simulink model "gm_hdl_generation_2"  (R2024b)
settings: Solver=VariableStepAuto  StartTime=0.0  StopTime=10.0  RelTol=1e-3
libraries: hdlmdlgenlib x4
settings Model: Creator=keybo  LastModifiedBy=keybo
settings OptimizationCC: BlockReduction=off  ConditionallyExecuteInputs=off  UseFloatMulNetSlope=on  InheritOutputTypeSmallerThanSingle=on  DefaultUnderspecifiedDataType=single
settings DebuggingCC: InheritedTsInSrcMsg=none

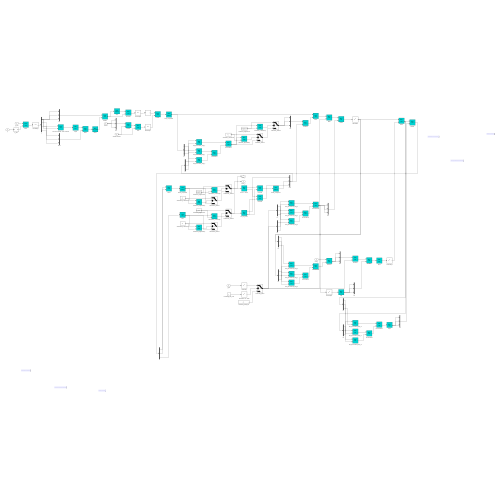
[thumbnail: Simulink's stored preview of the top-level diagram]
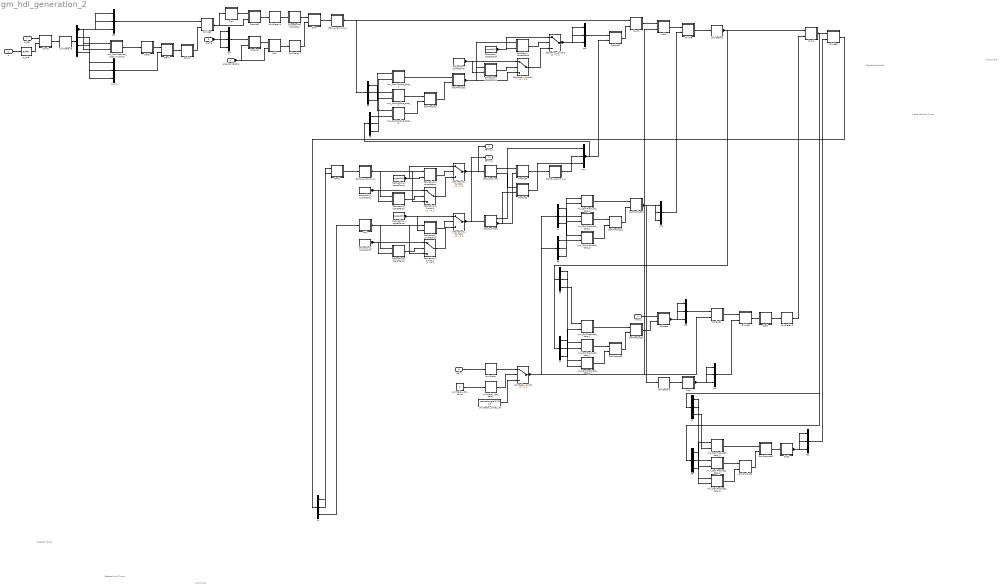
== system gm_hdl_generation_2 ==
  note: Attitude Controller
  note: Perpendicular Thrust
  note: Parallel Thrust
  note: Desired Unit Thrust
  note: Input to PID
  note: Unit Thrust
  q_des : Inport  OutDataTypeStr=single  PortDimensions=[4]  SampleTime=0.001
  q : Inport  Port=2  OutDataTypeStr=single  PortDimensions=[4]  SampleTime=0.001
  Inertia : Inport  Port=3  OutDataTypeStr=single  PortDimensions=1  SampleTime=0.001
  Angular Velocity : Inport  Port=4  OutDataTypeStr=single  PortDimensions=[3]  SampleTime=0.001
  r_gim : Inport  Port=5  OutDataTypeStr=single  PortDimensions=[3]  SampleTime=0.001
  norm_t : Inport  Port=6  OutDataTypeStr=single  PortDimensions=1  SampleTime=0.001
  Add : Subsystem
      mask Display: disp('NFP\nadd');
  Add1 : Subsystem
      mask Display: disp('NFP\nadd');
  Asin : Subsystem
      mask Display: disp('NFP\ntrig');
  Atan1 : Subsystem
      mask Display: disp('NFP\ntrig3');
  Atan2 : Subsystem
      mask Display: disp('NFP\ntrig3');
  Cos1_to_sincos : Subsystem
      mask Display: disp('NFP\ntrig2');
  Cos_to_sincos : Subsystem
      mask Display: disp('NFP\ntrig2');
  Discrete PID Controller : Subsystem
  Divide : Subsystem
      mask Display: disp('NFP\nmul');
  Divide1 : Subsystem
      mask Display: disp('NFP\nmul');
  Divide2 : Subsystem
      mask Display: disp('NFP\nmul');
  Divide3 : Subsystem
      mask Display: disp('NFP\nmul');
  Dot Product : Subsystem
      mask Display: disp('NFP\nadd');
  Dot Product1 : Subsystem
      mask Display: disp('NFP\nadd');
  Dot Product11 : Subsystem
      mask Display: disp('NFP\nadd');
  Dot Product12 : Subsystem
      mask Display: disp('NFP\nadd');
  Dot Product2 : Subsystem
      mask Display: disp('NFP\nadd');
  Dot Product21 : Subsystem
      mask Display: disp('NFP\nadd');
  Dot Product3 : Subsystem
      mask Display: disp('NFP\nadd');
  Dot Product31 : Subsystem
      mask Display: disp('NFP\nadd');
  Gain1 : Subsystem
      mask Display: disp('NFP\ngain_pow2');
  Gain2_unaryminus : Subsystem
      mask Display: disp('NFP\numinus');
  Gain3_unaryminus : Subsystem
      mask Display: disp('NFP\numinus');
  Gain_unaryminus : Subsystem
      mask Display: disp('NFP\numinus');
  Product : Subsystem
      mask Display: disp('NFP\nmul');
  Product1 : Subsystem
      mask Display: disp('NFP\nmul');
  Product2 : Subsystem
      mask Display: disp('NFP\nmul');
  Product3 : Subsystem
      mask Display: disp('NFP\nmul');
  Product4 : Subsystem
      mask Display: disp('NFP\nmul');
  Product5 : Subsystem
      mask Display: disp('NFP\nmul');
  Saturation1_LowerConst : Constant  Value=single(-0.5)  OutDataTypeStr=single  SampleTime=0.001
  Saturation1_LowerRelop : Subsystem
      mask Display: disp('NFP\nrelop');
  Saturation1_Switch1 : Switch  Criteria=u2 ~= 0  Threshold=double(0)  OutDataTypeStr=single  SampleTime=0.001  SaturateOnIntegerOverflow=off  InputSameDT=off
  Saturation1_Switch2 : Switch  Criteria=u2 ~= 0  Threshold=double(0)  OutDataTypeStr=single  SampleTime=0.001  SaturateOnIntegerOverflow=off  InputSameDT=off
  Saturation1_UpperConst : Constant  Value=single(0.5)  OutDataTypeStr=single  SampleTime=0.001
  Saturation1_UpperRelop : Subsystem
      mask Display: disp('NFP\nrelop');
  Saturation2_LowerConst : Constant  Value=single(-0.5)  OutDataTypeStr=single  SampleTime=0.001
  Saturation2_LowerRelop : Subsystem
      mask Display: disp('NFP\nrelop');
  Saturation2_Switch1 : Switch  Criteria=u2 ~= 0  Threshold=double(0)  OutDataTypeStr=single  SampleTime=0.001  SaturateOnIntegerOverflow=off  InputSameDT=off
  Saturation2_Switch2 : Switch  Criteria=u2 ~= 0  Threshold=double(0)  OutDataTypeStr=single  SampleTime=0.001  SaturateOnIntegerOverflow=off  InputSameDT=off
  Saturation2_UpperConst : Constant  Value=single(0.5)  OutDataTypeStr=single  SampleTime=0.001
  Saturation2_UpperRelop : Subsystem
      mask Display: disp('NFP\nrelop');
  Saturation_LowerConst : Constant  Value=single(-0.5)  OutDataTypeStr=single  SampleTime=0.001
  Saturation_LowerRelop : Subsystem
      mask Display: disp('NFP\nrelop');
  Saturation_Switch1 : Switch  Criteria=u2 ~= 0  Threshold=double(0)  OutDataTypeStr=single  SampleTime=0.001  SaturateOnIntegerOverflow=off  InputSameDT=off
  Saturation_Switch2 : Switch  Criteria=u2 ~= 0  Threshold=double(0)  OutDataTypeStr=single  SampleTime=0.001  SaturateOnIntegerOverflow=off  InputSameDT=off
  Saturation_UpperConst : Constant  Value=single(0.5)  OutDataTypeStr=single  SampleTime=0.001
  Saturation_UpperRelop : Subsystem
      mask Display: disp('NFP\nrelop');
  Sign : Subsystem
      mask Display: disp('NFP\nsignum');
  Sqrt : Subsystem
      mask Display: disp('NFP\nsqrt');
  Sqrt1 : Subsystem
      mask Display: disp('NFP\nsqrt');
  Sqrt2 : Subsystem
      mask Display: disp('NFP\nsqrt');
  Sqrt3 : Subsystem
      mask Display: disp('NFP\nsqrt');
  Subtract : Subsystem
      mask Display: disp('NFP\nadd');
  Sum : Subsystem
      mask Display: disp('NFP\nadd');
  Sum1 : Subsystem
      mask Display: disp('NFP\nadd');
  Sum2 : Subsystem
      mask Display: disp('NFP\nadd');
  Sum3 : Subsystem
      mask Display: disp('NFP\nadd');
  Unit Delay{,1..3,5..7} (7 alike) : Delay  DelayLength=double(1)  InitialCondition=0  SampleTime=0.001
  Unit Delay_Initial_Val : Constant  Value="repmat(single(1),[3  1])"  OutDataTypeStr=single  SampleTime=0.001
  Unit Delay_ctrl_const : Constant  OutDataTypeStr=boolean  SampleTime=0.001
  Unit Delay_ctrl_delay : Delay  DelayLength=double(1)  InitialCondition=0  SampleTime=0.001
  Unit Delay_switch : Switch  Criteria=u2 ~= 0  Threshold=double(0)  OutDataTypeStr=single  SampleTime=0.001  SaturateOnIntegerOverflow=off  InputSameDT=off
  mul_Dot Product1_dotp_0 : Subsystem
      mask Display: disp('NFP\nmul');
  mul_Dot Product1_dotp_1 : Subsystem
      mask Display: disp('NFP\nmul');
  mul_Dot Product1_dotp_2 : Subsystem
      mask Display: disp('NFP\nmul');
  mul_Dot Product2_dotp_0 : Subsystem
      mask Display: disp('NFP\nmul');
  mul_Dot Product2_dotp_1 : Subsystem
      mask Display: disp('NFP\nmul');
  mul_Dot Product2_dotp_2 : Subsystem
      mask Display: disp('NFP\nmul');
  mul_Dot Product3_dotp_0 : Subsystem
      mask Display: disp('NFP\nmul');
  mul_Dot Product3_dotp_1 : Subsystem
      mask Display: disp('NFP\nmul');
  mul_Dot Product3_dotp_2 : Subsystem
      mask Display: disp('NFP\nmul');
  mul_Dot Product4_dotp_mulcomp : Subsystem
      mask Display: disp('NFP\nmul');
  mul_Dot Product_dotp_0 : Subsystem
      mask Display: disp('NFP\nmul');
  mul_Dot Product_dotp_1 : Subsystem
      mask Display: disp('NFP\nmul');
  mul_Dot Product_dotp_2 : Subsystem
      mask Display: disp('NFP\nmul');
  mux : Mux  Inputs=3
  mux1 : Mux  Inputs=3
  q_wire : hdlmdlgenlib/Buffer
  t : Demux
  t{1..9} (9 alike) : Demux  Outputs=3
  t{10..16} (7 alike) : Mux  Inputs=3
  servo_x : Outport  SampleTime=0.001  VectorParamsAs1DForOutWhenUnconnected=off
  servo_y : Outport  Port=2  SampleTime=0.001  VectorParamsAs1DForOutWhenUnconnected=off
  wires:
  mul_Dot Product1_dotp_1/1(Out1) -> Dot Product11/1(In1)
  Dot Product31/1(Out1) -> Sqrt2/1(In1)
  t/3 -> mux1/2
  Saturation1_LowerRelop/1(Out1) -> Saturation1_Switch2/2
  Product3/1(Out1) -> Unit Delay6/1
  Unit Delay_switch/1 -> t4/1, t5/1, Product1/2(In2), Add1/2(In2)
  Discrete PID Controller/1(y) -> Sum/1(In1)
  Sqrt/1(Out1) -> t11/1, t11/2, t11/3
  t2/1 -> mul_Dot Product_dotp_0/1(In1)
  r_gim/1 -> Unit Delay/1
  Divide3/1(Out1) -> Sign/1(In1), Product3/2(In2)
  Dot Product2/1(Out1) -> Dot Product21/2(In2)
  Saturation2_UpperRelop/1(Out1) -> Saturation2_Switch1/2
  t2/3 -> mul_Dot Product_dotp_2/1(In1)
  Unit Delay_ctrl_delay/1 -> Unit Delay_switch/2
  t4/2 -> mul_Dot Product1_dotp_1/1(In1)
  Unit Delay_ctrl_const/1 -> Unit Delay_ctrl_delay/1
  t6/3 -> mul_Dot Product2_dotp_2/1(In1)
  Saturation2_UpperConst/1 -> Saturation2_LowerRelop/2(In2), Saturation2_Switch2/1
  mul_Dot Product2_dotp_1/1(Out1) -> Dot Product2/1(In1)
  Saturation2_LowerConst/1 -> Saturation2_UpperRelop/2(In2), Saturation2_Switch1/1
  Unit Delay3/1 -> Sum1/2(In2)
  Cos_to_sincos/1(Out1) -> mux/1
  t1/1 -> Atan2/1(In1)
  Unit Delay_Initial_Val/1 -> Unit Delay_switch/3
  t2/2 -> mul_Dot Product_dotp_1/1(In1)
  t1/2 -> Atan2/2(In2)
  t/4 -> mux1/3
  Cos_to_sincos/2(Out2) -> Product5/2(In2), Product4/2(In2)
  Dot Product11/1(Out1) -> Dot Product12/2(In2)
  mul_Dot Product3_dotp_0/1(Out1) -> Dot Product3/2(In2)
  Unit Delay2/1 -> Sqrt/1(In1)
  t/2 -> mux1/1
  t3/1 -> mul_Dot Product_dotp_0/2(In2)
  Sum2/1(Out1) -> Add1/1(In1)
  t4/3 -> mul_Dot Product1_dotp_2/1(In1)
  q_wire/1 -> Sum3/2(In2)
  Saturation1_Switch2/1 -> Cos1_to_sincos/1(In1), servo_x/1
  Sign/1(Out1) -> Product3/1(In1)
  Inertia/1 -> t14/1, t14/2, t14/3
  Dot Product12/1(Out1) -> t10/2, Unit Delay2/1, t10/1, t10/3
  Sum1/1(Out1) -> Divide2/1(In1), t9/1, t8/1
  t3/3 -> mul_Dot Product_dotp_2/2(In2)
  t3/2 -> mul_Dot Product_dotp_1/2(In2)
  t5/1 -> mul_Dot Product1_dotp_0/2(In2)
  t4/1 -> mul_Dot Product1_dotp_0/1(In1)
  Product5/1(Out1) -> mux/3
  t11/1 -> Divide1/2(In2)
  Sqrt3/1(Out1) -> Atan1/1(In1)
  norm_t/1 -> Subtract/1(In1)
  mul_Dot Product_dotp_2/1(Out1) -> Dot Product1/1(In1)
  Unit Delay1/1 -> Sum1/1(In1), t7/1, t6/1
  mul_Dot Product3_dotp_1/1(Out1) -> Dot Product3/1(In1)
  t8/2 -> mul_Dot Product3_dotp_1/1(In1)
  Add/1(Out1) -> Unit Delay7/1
  mul_Dot Product1_dotp_2/1(Out1) -> Dot Product12/1(In1)
  t16/1 -> Product2/1(In1)
  Sqrt2/1(Out1) -> t12/1, t12/2, t12/3
  Saturation_UpperConst/1 -> Saturation_LowerRelop/2(In2), Saturation_Switch2/1
  Saturation1_Switch1/1 -> Saturation1_Switch2/3
  Dot Product1/1(Out1) -> Saturation_Switch1/3, Saturation_UpperRelop/1(In1), Saturation_LowerRelop/1(In1)
  Gain_unaryminus/1(Out1) -> t2/1, Sum2/1(In1)
  Saturation_Switch1/1 -> Saturation_Switch2/3
  Angular Velocity/1 -> Product/2(In2), Add/2(In2)
  mul_Dot Product2_dotp_2/1(Out1) -> Dot Product21/1(In1)
  Saturation1_LowerConst/1 -> Saturation1_UpperRelop/2(In2), Saturation1_Switch1/1
  t1/3 -> Asin/1(In1)
  t6/2 -> mul_Dot Product2_dotp_1/1(In1)
  Sum3/1(Out1) -> Unit Delay5/1
  mux1/1 -> Atan1/2(In2)
  q/1 -> q_wire/1
  t8/3 -> mul_Dot Product3_dotp_2/1(In1)
  mux/1 -> Product2/2(In2), t3/1
  Gain2_unaryminus/1(Out1) -> Saturation1_UpperRelop/1(In1), Saturation1_LowerRelop/1(In1), Saturation1_Switch1/3
  t9/1 -> mul_Dot Product3_dotp_0/2(In2)
  Dot Product3/1(Out1) -> Dot Product31/2(In2)
  Asin/1(Out1) -> Saturation2_UpperRelop/1(In1), Saturation2_Switch1/3, Saturation2_LowerRelop/1(In1)
  Saturation1_UpperConst/1 -> Saturation1_LowerRelop/2(In2), Saturation1_Switch2/1
  Unit Delay7/1 -> Sum/2(In2)
  Saturation2_LowerRelop/1(Out1) -> Saturation2_Switch2/2
  Product2/1(Out1) -> Sum2/2(In2)
  Cos1_to_sincos/1(Out1) -> Product4/1(In1)
  Unit Delay5/1 -> t/1
  Divide1/1(Out1) -> Sqrt1/1(In1)
  Atan1/1(Out1) -> Gain1/1(In1)
  mul_Dot Product_dotp_1/1(Out1) -> Dot Product/1(In1)
  Gain3_unaryminus/1(Out1) -> mux/2
  Saturation2_Switch2/1 -> servo_y/1, Cos_to_sincos/1(In1)
  Gain1/1(Out1) -> Divide3/2(In2)
  mul_Dot Product4_dotp_mulcomp/1(Out1) -> Sqrt3/1(In1)
  Saturation_LowerConst/1 -> Saturation_UpperRelop/2(In2), Saturation_Switch1/1
  t5/3 -> mul_Dot Product1_dotp_2/2(In2)
  mul_Dot Product3_dotp_2/1(Out1) -> Dot Product31/1(In1)
  t14/1 -> Product/1(In1)
  mul_Dot Product_dotp_0/1(Out1) -> Dot Product/2(In2)
  Saturation2_Switch1/1 -> Saturation2_Switch2/3
  t8/1 -> mul_Dot Product3_dotp_0/1(In1)
  q_des/1 -> Sum3/1(In1)
  Dot Product21/1(Out1) -> Subtract/2(In2)
  Sum/1(Out1) -> Gain_unaryminus/1(In1)
  t9/3 -> mul_Dot Product3_dotp_2/2(In2)
  t/1 -> mul_Dot Product4_dotp_mulcomp/1(In1), t13/2, t13/1, t13/3, mul_Dot Product4_dotp_mulcomp/2(In2)
  Dot Product/1(Out1) -> Dot Product1/2(In2)
  t13/1 -> Divide3/1(In1)
  Saturation1_UpperRelop/1(Out1) -> Saturation1_Switch1/2
  t6/1 -> mul_Dot Product2_dotp_0/1(In1)
  Saturation_LowerRelop/1(Out1) -> Saturation_Switch2/2
  Divide2/1(Out1) -> t1/1
  Atan2/1(Out1) -> Gain2_unaryminus/1(In1)
  t9/2 -> mul_Dot Product3_dotp_1/2(In2)
  Product/1(Out1) -> Add/1(In1)
  Subtract/1(Out1) -> t15/1, t15/2, t15/3
  Cos1_to_sincos/2(Out2) -> Product5/1(In1)
  t5/2 -> mul_Dot Product1_dotp_1/2(In2)
  t7/2 -> mul_Dot Product2_dotp_1/2(In2)
  Unit Delay6/1 -> Discrete PID Controller/1(u)
  Saturation_Switch2/1 -> t16/1, t16/3, t16/2
  Sqrt1/1(Out1) -> Unit Delay3/1
  Product1/1(Out1) -> Divide1/1(In1)
  t7/1 -> mul_Dot Product2_dotp_0/2(In2)
  mul_Dot Product2_dotp_0/1(Out1) -> Dot Product2/2(In2)
  Unit Delay/1 -> Unit Delay_switch/1
  Divide/1(Out1) -> Unit Delay1/1
  t10/1 -> Divide/2(In2)
  t7/3 -> mul_Dot Product2_dotp_2/2(In2)
  Add1/1(Out1) -> Divide/1(In1)
  Saturation_UpperRelop/1(Out1) -> Saturation_Switch1/2
  t12/1 -> Divide2/2(In2)
  t15/1 -> Product1/1(In1)
  mul_Dot Product1_dotp_0/1(Out1) -> Dot Product11/2(In2)
  Product4/1(Out1) -> Gain3_unaryminus/1(In1)

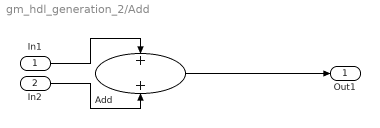
== system gm_hdl_generation_2/Add ==
  In1 : Inport
  In2 : Inport  Port=2
  Add : Sum  OutDataTypeStr=single  SampleTime=0.001
  Out1 : Outport
  wires:
  In1/1 -> Add/1
  In2/1 -> Add/2
  Add/1 -> Out1/1

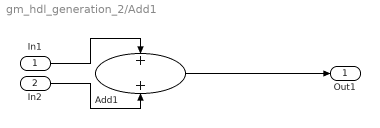
== system gm_hdl_generation_2/Add1 ==
  In1 : Inport
  In2 : Inport  Port=2
  Add1 : Sum  OutDataTypeStr=single  SampleTime=0.001
  Out1 : Outport
  wires:
  In1/1 -> Add1/1
  In2/1 -> Add1/2
  Add1/1 -> Out1/1

== system gm_hdl_generation_2/Asin ==
  In1 : Inport
  Asin : Trigonometry  Operator=asin  SampleTime=0.001
  Out1 : Outport
  wires:
  In1/1 -> Asin/1
  Asin/1 -> Out1/1

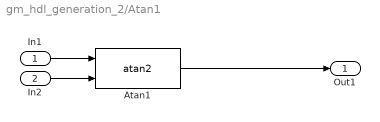
== system gm_hdl_generation_2/Atan1 ==
  In1 : Inport
  In2 : Inport  Port=2
  Atan1 : Trigonometry  Operator=atan2  SampleTime=0.001
  Out1 : Outport
  wires:
  In1/1 -> Atan1/1
  In2/1 -> Atan1/2
  Atan1/1 -> Out1/1

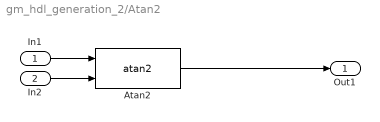
== system gm_hdl_generation_2/Atan2 ==
  In1 : Inport
  In2 : Inport  Port=2
  Atan2 : Trigonometry  Operator=atan2  SampleTime=0.001
  Out1 : Outport
  wires:
  In1/1 -> Atan2/1
  In2/1 -> Atan2/2
  Atan2/1 -> Out1/1

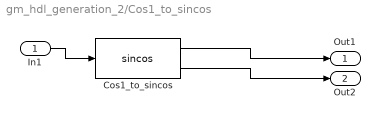
== system gm_hdl_generation_2/Cos1_to_sincos ==
  In1 : Inport
  Cos1_to_sincos : Trigonometry  Operator=sincos  SampleTime=0.001
  Out1 : Outport
  Out2 : Outport  Port=2
  wires:
  In1/1 -> Cos1_to_sincos/1
  Cos1_to_sincos/1 -> Out1/1
  Cos1_to_sincos/2 -> Out2/1

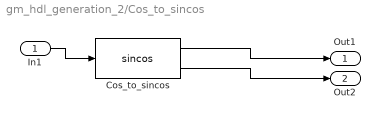
== system gm_hdl_generation_2/Cos_to_sincos ==
  In1 : Inport
  Cos_to_sincos : Trigonometry  Operator=sincos  SampleTime=0.001
  Out1 : Outport
  Out2 : Outport  Port=2
  wires:
  In1/1 -> Cos_to_sincos/1
  Cos_to_sincos/1 -> Out1/1
  Cos_to_sincos/2 -> Out2/1

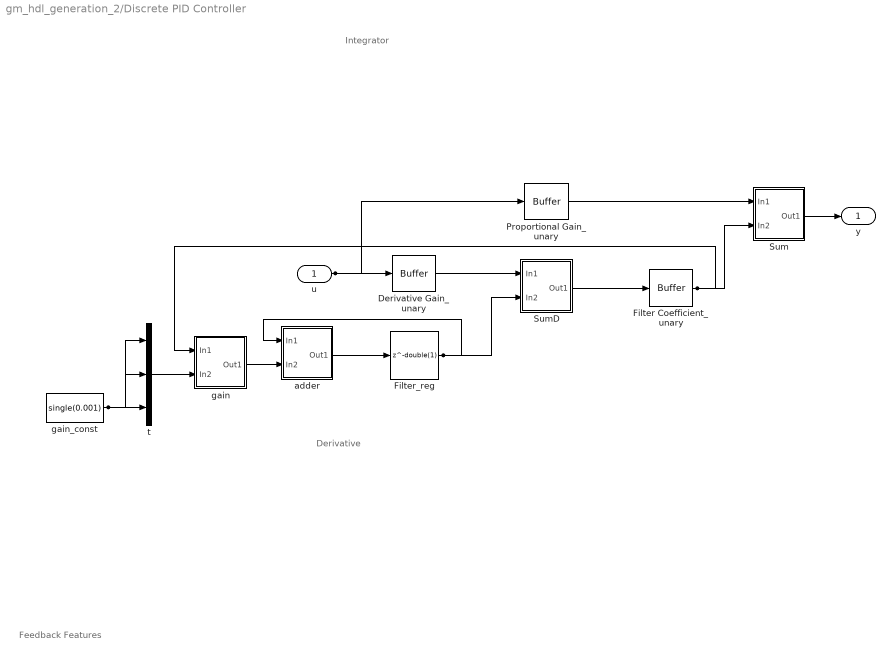
== system gm_hdl_generation_2/Discrete PID Controller ==
  note: Integrator
  note: Derivative
  note: Feedback Features
  u : Inport  OutDataTypeStr=single  PortDimensions=[3]  SampleTime=0.001
  Derivative Gain_unary : hdlmdlgenlib/Buffer
  Filter Coefficient_unary : hdlmdlgenlib/Buffer
  Filter_reg : Delay  DelayLength=double(1)  InitialCondition=0  SampleTime=0.001
  Proportional Gain_unary : hdlmdlgenlib/Buffer
  Sum : Subsystem
      mask Display: disp('NFP\nadd');
  SumD : Subsystem
      mask Display: disp('NFP\nadd');
  adder : Subsystem
      mask Display: disp('NFP\nadd');
  gain : Subsystem
      mask Display: disp('NFP\nmul');
  gain_const : Constant  Value=single(0.001)  OutDataTypeStr=single  SampleTime=0.001
  t : Mux  Inputs=3
  y : Outport  SampleTime=0.001
  wires:
  Filter Coefficient_unary/1 -> Sum/2(In2), gain/1(In1)
  Proportional Gain_unary/1 -> Sum/1(In1)
  Filter_reg/1 -> SumD/2(In2), adder/1(In1)
  Derivative Gain_unary/1 -> SumD/1(In1)
  adder/1(Out1) -> Filter_reg/1
  gain/1(Out1) -> adder/2(In2)
  SumD/1(Out1) -> Filter Coefficient_unary/1
  t/1 -> gain/2(In2)
  Sum/1(Out1) -> y/1
  u/1 -> Derivative Gain_unary/1, Proportional Gain_unary/1
  gain_const/1 -> t/1, t/2, t/3

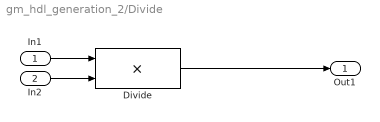
== system gm_hdl_generation_2/Divide ==
  In1 : Inport
  In2 : Inport  Port=2
  Divide : Product  Inputs=**  OutDataTypeStr=single  SampleTime=0.001
  Out1 : Outport
  wires:
  In1/1 -> Divide/1
  In2/1 -> Divide/2
  Divide/1 -> Out1/1

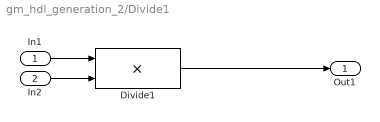
== system gm_hdl_generation_2/Divide1 ==
  In1 : Inport
  In2 : Inport  Port=2
  Divide1 : Product  Inputs=**  OutDataTypeStr=single  SampleTime=0.001
  Out1 : Outport
  wires:
  In1/1 -> Divide1/1
  In2/1 -> Divide1/2
  Divide1/1 -> Out1/1

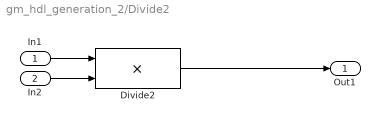
== system gm_hdl_generation_2/Divide2 ==
  In1 : Inport
  In2 : Inport  Port=2
  Divide2 : Product  Inputs=**  OutDataTypeStr=single  SampleTime=0.001
  Out1 : Outport
  wires:
  In1/1 -> Divide2/1
  In2/1 -> Divide2/2
  Divide2/1 -> Out1/1

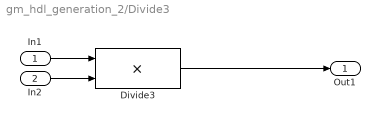
== system gm_hdl_generation_2/Divide3 ==
  In1 : Inport
  In2 : Inport  Port=2
  Divide3 : Product  Inputs=**  OutDataTypeStr=single  SampleTime=0.001
  Out1 : Outport
  wires:
  In1/1 -> Divide3/1
  In2/1 -> Divide3/2
  Divide3/1 -> Out1/1

== system gm_hdl_generation_2/Dot Product ==
  In1 : Inport
  In2 : Inport  Port=2
  Dot Product : Sum  OutDataTypeStr=single  SampleTime=0.001
  Out1 : Outport
  wires:
  In1/1 -> Dot Product/1
  In2/1 -> Dot Product/2
  Dot Product/1 -> Out1/1

== system gm_hdl_generation_2/Dot Product1 ==
  In1 : Inport
  In2 : Inport  Port=2
  Dot Product1 : Sum  OutDataTypeStr=single  SampleTime=0.001
  Out1 : Outport
  wires:
  In1/1 -> Dot Product1/1
  In2/1 -> Dot Product1/2
  Dot Product1/1 -> Out1/1

== system gm_hdl_generation_2/Dot Product11 ==
  In1 : Inport
  In2 : Inport  Port=2
  Dot Product11 : Sum  OutDataTypeStr=single  SampleTime=0.001
  Out1 : Outport
  wires:
  In1/1 -> Dot Product11/1
  In2/1 -> Dot Product11/2
  Dot Product11/1 -> Out1/1

== system gm_hdl_generation_2/Dot Product12 ==
  In1 : Inport
  In2 : Inport  Port=2
  Dot Product12 : Sum  OutDataTypeStr=single  SampleTime=0.001
  Out1 : Outport
  wires:
  In1/1 -> Dot Product12/1
  In2/1 -> Dot Product12/2
  Dot Product12/1 -> Out1/1

== system gm_hdl_generation_2/Dot Product2 ==
  In1 : Inport
  In2 : Inport  Port=2
  Dot Product2 : Sum  OutDataTypeStr=single  SampleTime=0.001
  Out1 : Outport
  wires:
  In1/1 -> Dot Product2/1
  In2/1 -> Dot Product2/2
  Dot Product2/1 -> Out1/1

== system gm_hdl_generation_2/Dot Product21 ==
  In1 : Inport
  In2 : Inport  Port=2
  Dot Product21 : Sum  OutDataTypeStr=single  SampleTime=0.001
  Out1 : Outport
  wires:
  In1/1 -> Dot Product21/1
  In2/1 -> Dot Product21/2
  Dot Product21/1 -> Out1/1

== system gm_hdl_generation_2/Dot Product3 ==
  In1 : Inport
  In2 : Inport  Port=2
  Dot Product3 : Sum  OutDataTypeStr=single  SampleTime=0.001
  Out1 : Outport
  wires:
  In1/1 -> Dot Product3/1
  In2/1 -> Dot Product3/2
  Dot Product3/1 -> Out1/1

== system gm_hdl_generation_2/Dot Product31 ==
  In1 : Inport
  In2 : Inport  Port=2
  Dot Product31 : Sum  OutDataTypeStr=single  SampleTime=0.001
  Out1 : Outport
  wires:
  In1/1 -> Dot Product31/1
  In2/1 -> Dot Product31/2
  Dot Product31/1 -> Out1/1

== system gm_hdl_generation_2/Gain1 ==
  In1 : Inport
  Gain1 : Gain  Gain=single(2)
  Out1 : Outport
  wires:
  In1/1 -> Gain1/1
  Gain1/1 -> Out1/1

== system gm_hdl_generation_2/Gain2_unaryminus ==
  In1 : Inport
  Gain2_unaryminus : UnaryMinus  SampleTime=0.001
  Out1 : Outport
  wires:
  In1/1 -> Gain2_unaryminus/1
  Gain2_unaryminus/1 -> Out1/1

== system gm_hdl_generation_2/Gain3_unaryminus ==
  In1 : Inport
  Gain3_unaryminus : UnaryMinus  SampleTime=0.001
  Out1 : Outport
  wires:
  In1/1 -> Gain3_unaryminus/1
  Gain3_unaryminus/1 -> Out1/1

== system gm_hdl_generation_2/Gain_unaryminus ==
  In1 : Inport
  Gain_unaryminus : UnaryMinus  SampleTime=0.001
  Out1 : Outport
  wires:
  In1/1 -> Gain_unaryminus/1
  Gain_unaryminus/1 -> Out1/1

== system gm_hdl_generation_2/Product ==
  In1 : Inport
  In2 : Inport  Port=2
  Product : Product  Inputs=**  OutDataTypeStr=single  SampleTime=0.001
  Out1 : Outport
  wires:
  In1/1 -> Product/1
  In2/1 -> Product/2
  Product/1 -> Out1/1

== system gm_hdl_generation_2/Product1 ==
  In1 : Inport
  In2 : Inport  Port=2
  Product1 : Product  Inputs=**  OutDataTypeStr=single  SampleTime=0.001
  Out1 : Outport
  wires:
  In1/1 -> Product1/1
  In2/1 -> Product1/2
  Product1/1 -> Out1/1

== system gm_hdl_generation_2/Product2 ==
  In1 : Inport
  In2 : Inport  Port=2
  Product2 : Product  Inputs=**  OutDataTypeStr=single  SampleTime=0.001
  Out1 : Outport
  wires:
  In1/1 -> Product2/1
  In2/1 -> Product2/2
  Product2/1 -> Out1/1

== system gm_hdl_generation_2/Product3 ==
  In1 : Inport
  In2 : Inport  Port=2
  Product3 : Product  Inputs=**  OutDataTypeStr=single  SampleTime=0.001
  Out1 : Outport
  wires:
  In1/1 -> Product3/1
  In2/1 -> Product3/2
  Product3/1 -> Out1/1

== system gm_hdl_generation_2/Product4 ==
  In1 : Inport
  In2 : Inport  Port=2
  Product4 : Product  Inputs=**  OutDataTypeStr=single  SampleTime=0.001
  Out1 : Outport
  wires:
  In1/1 -> Product4/1
  In2/1 -> Product4/2
  Product4/1 -> Out1/1

== system gm_hdl_generation_2/Product5 ==
  In1 : Inport
  In2 : Inport  Port=2
  Product5 : Product  Inputs=**  OutDataTypeStr=single  SampleTime=0.001
  Out1 : Outport
  wires:
  In1/1 -> Product5/1
  In2/1 -> Product5/2
  Product5/1 -> Out1/1

== system gm_hdl_generation_2/Saturation1_LowerRelop ==
  In1 : Inport
  In2 : Inport  Port=2
  Saturation1_LowerRelop : RelationalOperator  Operator=>  OutDataTypeStr=boolean  SampleTime=0.001  InputSameDT=off
  Out1 : Outport
  wires:
  In1/1 -> Saturation1_LowerRelop/1
  In2/1 -> Saturation1_LowerRelop/2
  Saturation1_LowerRelop/1 -> Out1/1

== system gm_hdl_generation_2/Saturation1_UpperRelop ==
  In1 : Inport
  In2 : Inport  Port=2
  Saturation1_UpperRelop : RelationalOperator  Operator=<  OutDataTypeStr=boolean  SampleTime=0.001  InputSameDT=off
  Out1 : Outport
  wires:
  In1/1 -> Saturation1_UpperRelop/1
  In2/1 -> Saturation1_UpperRelop/2
  Saturation1_UpperRelop/1 -> Out1/1

== system gm_hdl_generation_2/Saturation2_LowerRelop ==
  In1 : Inport
  In2 : Inport  Port=2
  Saturation2_LowerRelop : RelationalOperator  Operator=>  OutDataTypeStr=boolean  SampleTime=0.001  InputSameDT=off
  Out1 : Outport
  wires:
  In1/1 -> Saturation2_LowerRelop/1
  In2/1 -> Saturation2_LowerRelop/2
  Saturation2_LowerRelop/1 -> Out1/1

== system gm_hdl_generation_2/Saturation2_UpperRelop ==
  In1 : Inport
  In2 : Inport  Port=2
  Saturation2_UpperRelop : RelationalOperator  Operator=<  OutDataTypeStr=boolean  SampleTime=0.001  InputSameDT=off
  Out1 : Outport
  wires:
  In1/1 -> Saturation2_UpperRelop/1
  In2/1 -> Saturation2_UpperRelop/2
  Saturation2_UpperRelop/1 -> Out1/1

== system gm_hdl_generation_2/Saturation_LowerRelop ==
  In1 : Inport
  In2 : Inport  Port=2
  Saturation_LowerRelop : RelationalOperator  Operator=>  OutDataTypeStr=boolean  SampleTime=0.001  InputSameDT=off
  Out1 : Outport
  wires:
  In1/1 -> Saturation_LowerRelop/1
  In2/1 -> Saturation_LowerRelop/2
  Saturation_LowerRelop/1 -> Out1/1

== system gm_hdl_generation_2/Saturation_UpperRelop ==
  In1 : Inport
  In2 : Inport  Port=2
  Saturation_UpperRelop : RelationalOperator  Operator=<  OutDataTypeStr=boolean  SampleTime=0.001  InputSameDT=off
  Out1 : Outport
  wires:
  In1/1 -> Saturation_UpperRelop/1
  In2/1 -> Saturation_UpperRelop/2
  Saturation_UpperRelop/1 -> Out1/1

== system gm_hdl_generation_2/Sign ==
  In1 : Inport
  Sign : Signum  SampleTime=0.001
  Out1 : Outport
  wires:
  In1/1 -> Sign/1
  Sign/1 -> Out1/1

== system gm_hdl_generation_2/Sqrt ==
  In1 : Inport
  Sqrt : Sqrt  SampleTime=0.001
  Out1 : Outport
  wires:
  In1/1 -> Sqrt/1
  Sqrt/1 -> Out1/1

== system gm_hdl_generation_2/Sqrt1 ==
  In1 : Inport
  Sqrt1 : Sqrt  SampleTime=0.001
  Out1 : Outport
  wires:
  In1/1 -> Sqrt1/1
  Sqrt1/1 -> Out1/1

== system gm_hdl_generation_2/Sqrt2 ==
  In1 : Inport
  Sqrt2 : Sqrt  SampleTime=0.001
  Out1 : Outport
  wires:
  In1/1 -> Sqrt2/1
  Sqrt2/1 -> Out1/1

== system gm_hdl_generation_2/Sqrt3 ==
  In1 : Inport
  Sqrt3 : Sqrt  SampleTime=0.001
  Out1 : Outport
  wires:
  In1/1 -> Sqrt3/1
  Sqrt3/1 -> Out1/1

== system gm_hdl_generation_2/Subtract ==
  In1 : Inport
  In2 : Inport  Port=2
  Subtract : Sum  Inputs=+-  OutDataTypeStr=single  SampleTime=0.001
  Out1 : Outport
  wires:
  In1/1 -> Subtract/1
  In2/1 -> Subtract/2
  Subtract/1 -> Out1/1

== system gm_hdl_generation_2/Sum ==
  In1 : Inport
  In2 : Inport  Port=2
  Sum : Sum  OutDataTypeStr=single  SampleTime=0.001
  Out1 : Outport
  wires:
  In1/1 -> Sum/1
  In2/1 -> Sum/2
  Sum/1 -> Out1/1

== system gm_hdl_generation_2/Sum1 ==
  In1 : Inport
  In2 : Inport  Port=2
  Sum1 : Sum  OutDataTypeStr=single  SampleTime=0.001
  Out1 : Outport
  wires:
  In1/1 -> Sum1/1
  In2/1 -> Sum1/2
  Sum1/1 -> Out1/1

== system gm_hdl_generation_2/Sum2 ==
  In1 : Inport
  In2 : Inport  Port=2
  Sum2 : Sum  Inputs=+-  OutDataTypeStr=single  SampleTime=0.001
  Out1 : Outport
  wires:
  In1/1 -> Sum2/1
  In2/1 -> Sum2/2
  Sum2/1 -> Out1/1

== system gm_hdl_generation_2/Sum3 ==
  In1 : Inport
  In2 : Inport  Port=2
  Sum3 : Sum  OutDataTypeStr=single  SampleTime=0.001
  Out1 : Outport
  wires:
  In1/1 -> Sum3/1
  In2/1 -> Sum3/2
  Sum3/1 -> Out1/1

== system gm_hdl_generation_2/mul_Dot Product1_dotp_0 ==
  In1 : Inport
  In2 : Inport  Port=2
  mul_Dot Product1_dotp_0 : Product  Inputs=**  OutDataTypeStr=single  SampleTime=0.001
  Out1 : Outport
  wires:
  In1/1 -> mul_Dot Product1_dotp_0/1
  In2/1 -> mul_Dot Product1_dotp_0/2
  mul_Dot Product1_dotp_0/1 -> Out1/1

== system gm_hdl_generation_2/mul_Dot Product1_dotp_1 ==
  In1 : Inport
  In2 : Inport  Port=2
  mul_Dot Product1_dotp_1 : Product  Inputs=**  OutDataTypeStr=single  SampleTime=0.001
  Out1 : Outport
  wires:
  In1/1 -> mul_Dot Product1_dotp_1/1
  In2/1 -> mul_Dot Product1_dotp_1/2
  mul_Dot Product1_dotp_1/1 -> Out1/1

== system gm_hdl_generation_2/mul_Dot Product1_dotp_2 ==
  In1 : Inport
  In2 : Inport  Port=2
  mul_Dot Product1_dotp_2 : Product  Inputs=**  OutDataTypeStr=single  SampleTime=0.001
  Out1 : Outport
  wires:
  In1/1 -> mul_Dot Product1_dotp_2/1
  In2/1 -> mul_Dot Product1_dotp_2/2
  mul_Dot Product1_dotp_2/1 -> Out1/1

== system gm_hdl_generation_2/mul_Dot Product2_dotp_0 ==
  In1 : Inport
  In2 : Inport  Port=2
  mul_Dot Product2_dotp_0 : Product  Inputs=**  OutDataTypeStr=single  SampleTime=0.001
  Out1 : Outport
  wires:
  In1/1 -> mul_Dot Product2_dotp_0/1
  In2/1 -> mul_Dot Product2_dotp_0/2
  mul_Dot Product2_dotp_0/1 -> Out1/1

== system gm_hdl_generation_2/mul_Dot Product2_dotp_1 ==
  In1 : Inport
  In2 : Inport  Port=2
  mul_Dot Product2_dotp_1 : Product  Inputs=**  OutDataTypeStr=single  SampleTime=0.001
  Out1 : Outport
  wires:
  In1/1 -> mul_Dot Product2_dotp_1/1
  In2/1 -> mul_Dot Product2_dotp_1/2
  mul_Dot Product2_dotp_1/1 -> Out1/1

== system gm_hdl_generation_2/mul_Dot Product2_dotp_2 ==
  In1 : Inport
  In2 : Inport  Port=2
  mul_Dot Product2_dotp_2 : Product  Inputs=**  OutDataTypeStr=single  SampleTime=0.001
  Out1 : Outport
  wires:
  In1/1 -> mul_Dot Product2_dotp_2/1
  In2/1 -> mul_Dot Product2_dotp_2/2
  mul_Dot Product2_dotp_2/1 -> Out1/1

== system gm_hdl_generation_2/mul_Dot Product3_dotp_0 ==
  In1 : Inport
  In2 : Inport  Port=2
  mul_Dot Product3_dotp_0 : Product  Inputs=**  OutDataTypeStr=single  SampleTime=0.001
  Out1 : Outport
  wires:
  In1/1 -> mul_Dot Product3_dotp_0/1
  In2/1 -> mul_Dot Product3_dotp_0/2
  mul_Dot Product3_dotp_0/1 -> Out1/1

== system gm_hdl_generation_2/mul_Dot Product3_dotp_1 ==
  In1 : Inport
  In2 : Inport  Port=2
  mul_Dot Product3_dotp_1 : Product  Inputs=**  OutDataTypeStr=single  SampleTime=0.001
  Out1 : Outport
  wires:
  In1/1 -> mul_Dot Product3_dotp_1/1
  In2/1 -> mul_Dot Product3_dotp_1/2
  mul_Dot Product3_dotp_1/1 -> Out1/1

== system gm_hdl_generation_2/mul_Dot Product3_dotp_2 ==
  In1 : Inport
  In2 : Inport  Port=2
  mul_Dot Product3_dotp_2 : Product  Inputs=**  OutDataTypeStr=single  SampleTime=0.001
  Out1 : Outport
  wires:
  In1/1 -> mul_Dot Product3_dotp_2/1
  In2/1 -> mul_Dot Product3_dotp_2/2
  mul_Dot Product3_dotp_2/1 -> Out1/1

== system gm_hdl_generation_2/mul_Dot Product4_dotp_mulcomp ==
  In1 : Inport
  In2 : Inport  Port=2
  mul_Dot Product4_dotp_mulcomp : Product  Inputs=**  OutDataTypeStr=single  SampleTime=0.001
  Out1 : Outport
  wires:
  In1/1 -> mul_Dot Product4_dotp_mulcomp/1
  In2/1 -> mul_Dot Product4_dotp_mulcomp/2
  mul_Dot Product4_dotp_mulcomp/1 -> Out1/1

== system gm_hdl_generation_2/mul_Dot Product_dotp_0 ==
  In1 : Inport
  In2 : Inport  Port=2
  mul_Dot Product_dotp_0 : Product  Inputs=**  OutDataTypeStr=single  SampleTime=0.001
  Out1 : Outport
  wires:
  In1/1 -> mul_Dot Product_dotp_0/1
  In2/1 -> mul_Dot Product_dotp_0/2
  mul_Dot Product_dotp_0/1 -> Out1/1

== system gm_hdl_generation_2/mul_Dot Product_dotp_1 ==
  In1 : Inport
  In2 : Inport  Port=2
  mul_Dot Product_dotp_1 : Product  Inputs=**  OutDataTypeStr=single  SampleTime=0.001
  Out1 : Outport
  wires:
  In1/1 -> mul_Dot Product_dotp_1/1
  In2/1 -> mul_Dot Product_dotp_1/2
  mul_Dot Product_dotp_1/1 -> Out1/1

== system gm_hdl_generation_2/mul_Dot Product_dotp_2 ==
  In1 : Inport
  In2 : Inport  Port=2
  mul_Dot Product_dotp_2 : Product  Inputs=**  OutDataTypeStr=single  SampleTime=0.001
  Out1 : Outport
  wires:
  In1/1 -> mul_Dot Product_dotp_2/1
  In2/1 -> mul_Dot Product_dotp_2/2
  mul_Dot Product_dotp_2/1 -> Out1/1

== system gm_hdl_generation_2/Discrete PID Controller/Sum ==
  In1 : Inport
  In2 : Inport  Port=2
  Sum : Sum  OutDataTypeStr=single  SampleTime=0.001
  Out1 : Outport
  wires:
  In1/1 -> Sum/1
  In2/1 -> Sum/2
  Sum/1 -> Out1/1

== system gm_hdl_generation_2/Discrete PID Controller/SumD ==
  In1 : Inport
  In2 : Inport  Port=2
  SumD : Sum  Inputs=+-  OutDataTypeStr=single  SampleTime=0.001
  Out1 : Outport
  wires:
  In1/1 -> SumD/1
  In2/1 -> SumD/2
  SumD/1 -> Out1/1

== system gm_hdl_generation_2/Discrete PID Controller/adder ==
  In1 : Inport
  In2 : Inport  Port=2
  adder : Sum  OutDataTypeStr=single  SampleTime=0.001
  Out1 : Outport
  wires:
  In1/1 -> adder/1
  In2/1 -> adder/2
  adder/1 -> Out1/1

== system gm_hdl_generation_2/Discrete PID Controller/gain ==
  In1 : Inport
  In2 : Inport  Port=2
  gain : Product  Inputs=**  OutDataTypeStr=single  SampleTime=0.001
  Out1 : Outport
  wires:
  In1/1 -> gain/1
  In2/1 -> gain/2
  gain/1 -> Out1/1
